simulink model "W06_2_turn"  (R2024b)
settings: Solver=FixedStepDiscrete  StartTime=0.0  StopTime=80  FixedStep=0.05  RelTol=1e-3
libraries: ros2lib x4
settings Model: Creator=admin  LastModifiedBy=admin

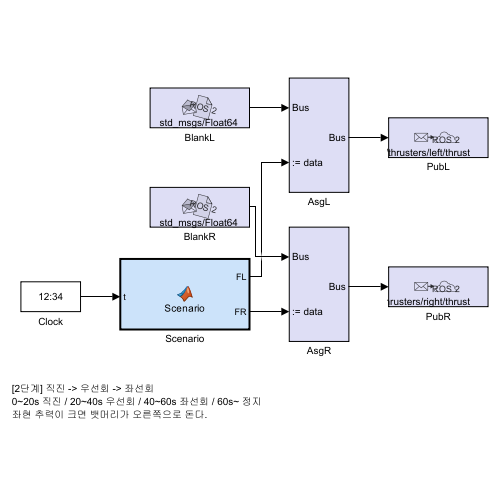
[thumbnail: Simulink's stored preview of the top-level diagram]
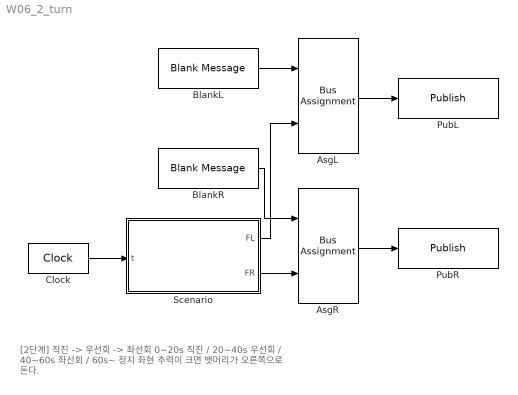
== system W06_2_turn ==
  note: [2단계] 직진 -> 우선회 -> 좌선회
      | 0~20s 직진 / 20~40s 우선회 / 40~60s 좌선회 / 60s~ 정지
      | 좌현 추력이 크면 뱃머리가 오른쪽으로 돈다.
  AsgL : BusAssignment  AssignedSignals=data
  AsgR : BusAssignment  AssignedSignals=data
  BlankL : ros2lib/Blank Message  messageClass=Message  entityType=std_msgs/Float64  messageType=std_msgs/Float64  SampleTime=0.05
  BlankR : ros2lib/Blank Message  messageClass=Message  entityType=std_msgs/Float64  messageType=std_msgs/Float64  SampleTime=0.05
  Clock : DigitalClock  SampleTime=0.05
  PubL : ros2lib/Publish  topicSource=Specify your own  topic=/wamv/thrusters/left/thrust  messageType=std_msgs/Float64  QOSHistory=Keep last  QOSDepth=1  QOSReliability=Reliable  QOSDurability=Volatile  QOSDeadline=Inf  QOSLifespan=Inf  QOSLiveliness=Automatic  QOSLeaseDuration=Inf  QOSAvoidROSNamespaceConventions=off
  PubR : ros2lib/Publish  topicSource=Specify your own  topic=/wamv/thrusters/right/thrust  messageType=std_msgs/Float64  QOSHistory=Keep last  QOSDepth=1  QOSReliability=Reliable  QOSDurability=Volatile  QOSDeadline=Inf  QOSLifespan=Inf  QOSLiveliness=Automatic  QOSLeaseDuration=Inf  QOSAvoidROSNamespaceConventions=off
  Scenario : MATLAB Function  TreatAsAtomicUnit=on
  wires:
  Scenario/2(FR) -> AsgR/2
  Scenario/1(FL) -> AsgL/2
  Clock/1 -> Scenario/1(t)
  AsgR/1 -> PubR/1
  BlankL/1 -> AsgL/1
  BlankR/1 -> AsgR/1
  AsgL/1 -> PubL/1

== matlab function W06_2_turn/Scenario ==
  data: t input; FL output; FR output
function [FL, FR] = Scenario(t)
%#codegen
% Time-based thrust scenario [N]
if t < 20
    FL = 200;  FR = 200;   % go straight
elseif t < 40
    FL = 300;  FR =  50;   % turn starboard (right)
elseif t < 60
    FL =  50;  FR = 300;   % turn port (left)
else
    FL = 0;    FR = 0;     % stop
end
